simulink model "RobustAdaptive_Control"  (R2022b)
settings: Solver=VariableStepAuto  StartTime=0.0  StopTime=60  RelTol=1e-3
settings Model: Creator=JianFongLee  LastModifiedBy=allen
settings DebuggingCC: UnconnectedInputMsg=warning  UnconnectedOutputMsg=warning  UnconnectedLineMsg=warning
settings ModelReferenceCC: EnableRefExpFcnMdlSchedulingChecks=on
settings RTWCC: DLArmComputeVersion=19.05

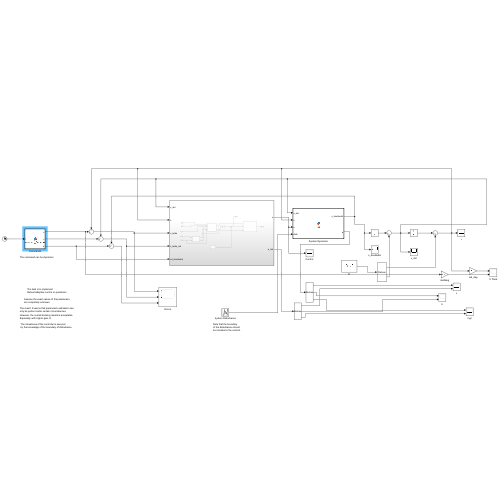
[thumbnail: Simulink's stored preview of the top-level diagram]
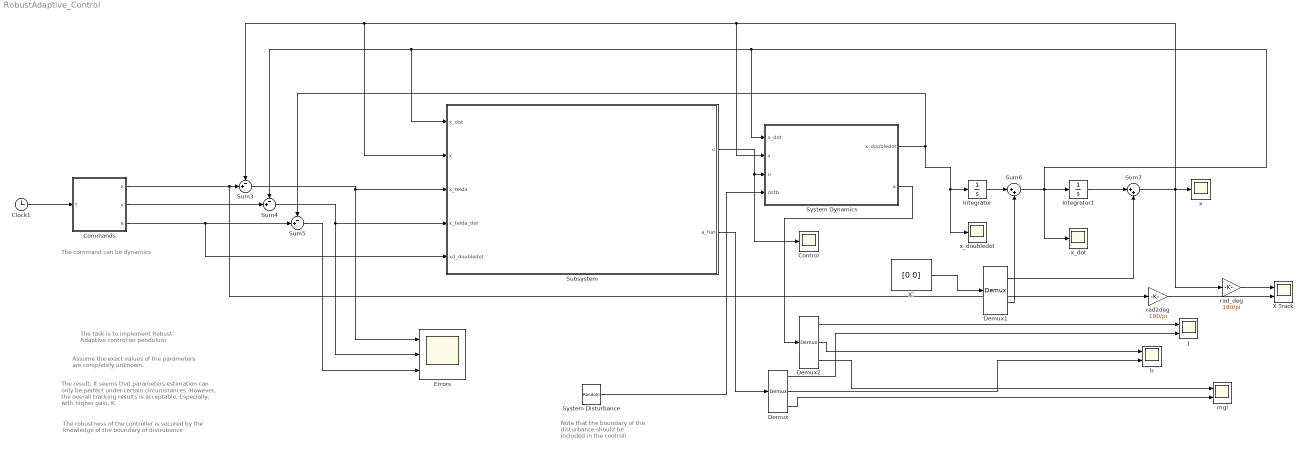
== system RobustAdaptive_Control ==
  note: The command can be dynamics
  note: The robustness of the controller is secured
      | by the knowledge of the boundary of distrubance
  note: Note that the boundary
      | of the disturbance should
      | be included in the controll.
  note: The result: It seems that parameters estimation can
      | only be perfect under certain circumstances.
      | However, the overall tracking results is acceptable.
      | Especially, with higher gain, K.
  note: Assume the exact values of the parameters
      | are completely unknown.
  note: The task is to implement
      | Robust Adaptive control on pendulum
  Clock1 : Clock
  Commands : MATLAB Function  TreatAsAtomicUnit=on
  Control : Scope
  Demux : Demux  Outputs=3
      settings: DisplayOption=none
  Demux1 : Demux  Outputs=2
      settings: DisplayOption=none
  Demux2 : Demux  Outputs=3
      settings: DisplayOption=none
  Errors : Scope  NumInputPorts=3
  IC : Constant  Value=[0 0]
  Integrator : Integrator
  Integrator1 : Integrator
  J : Scope  NumInputPorts=2
  Subsystem : Subsystem
  Sum3 : Sum  Inputs=-+|
  Sum4 : Sum  Inputs=-+|
  Sum5 : Sum  Inputs=-+|
  Sum6 : Sum  Inputs=|++
  Sum7 : Sum  Inputs=|++
  System Disturbance : UniformRandomNumber  Minimum=-2  Maximum=2  Seed=7
  System Dynamics : MATLAB Function  TreatAsAtomicUnit=on
  X Track : Scope  NumInputPorts=2
  b : Scope  NumInputPorts=2
  mgl : Scope  NumInputPorts=2
  rad2deg : Gain  Gain=180/pi
  rad_deg : Gain  Gain=180/pi
  x : Scope
  x_dot : Scope
  x_doubledot : Scope
  wires:
  Subsystem/1(u) -> Control/1, System Dynamics/3(u)
  IC/1 -> Demux1/1
  Integrator1/1 -> Sum7/1
  Integrator/1 -> Sum6/1
  Demux1/2 -> Sum6/2
  Sum6/1 -> x_dot/1, Subsystem/1(x_dot), Sum4/1, System Dynamics/1(x_dot), Integrator1/1
  Demux1/1 -> Sum7/2
  Sum7/1 -> rad_deg/1, Subsystem/2(x), Sum3/1, System Dynamics/2(x), x/1
  System Dynamics/1(x_doubledot) -> x_doubledot/1, Integrator/1, Sum5/1
  Sum3/1 -> Errors/1, Subsystem/3(x_telda)
  Sum4/1 -> Subsystem/4(x_telda_dot), Errors/2
  Clock1/1 -> Commands/1(t)
  Commands/1(x) -> rad2deg/1, Sum3/2
  Commands/2(v) -> Sum4/2
  Commands/3(a) -> Subsystem/5(xd_doubledot), Sum5/2
  Sum5/1 -> Errors/3
  Subsystem/2(a_hat) -> Demux/1
  System Dynamics/2(a) -> Demux2/1
  Demux2/1 -> J/1
  Demux/1 -> J/2
  Demux2/2 -> b/1
  Demux/2 -> b/2
  Demux2/3 -> mgl/1
  Demux/3 -> mgl/2
  rad_deg/1 -> X Track/1
  rad2deg/1 -> X Track/2
  System Disturbance/1 -> System Dynamics/4(dstb)

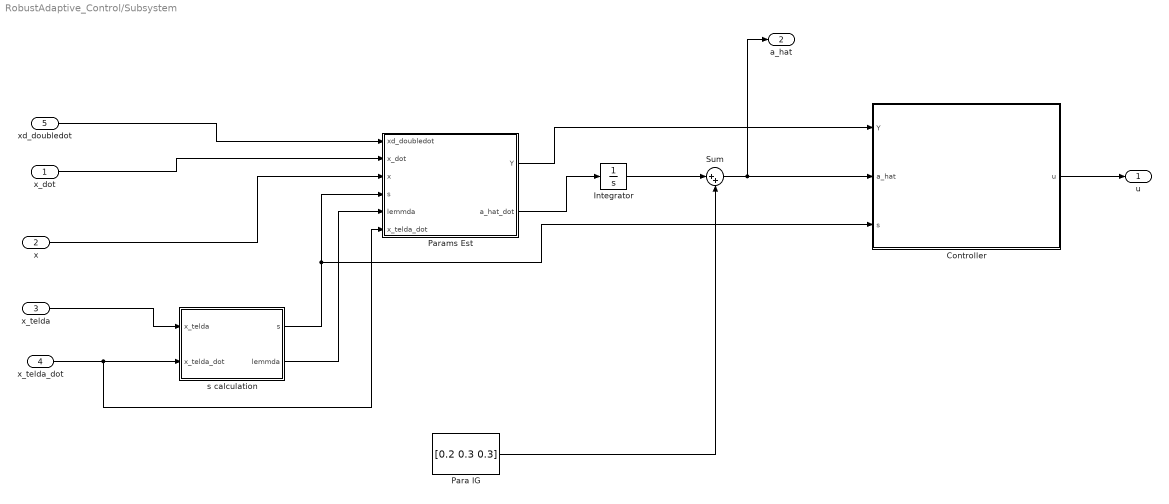
== system RobustAdaptive_Control/Subsystem ==
  x_dot : Inport
  x : Inport  Port=2
  x_telda : Inport  Port=3
  x_telda_dot : Inport  Port=4
  xd_doubledot : Inport  Port=5
  Controller : MATLAB Function  TreatAsAtomicUnit=on
  Integrator : Integrator
  Para IG : Constant  Value=[0.2 0.3 0.3]
  Params Est : MATLAB Function  TreatAsAtomicUnit=on
  Sum : Sum  Inputs=|++
  s calculation : MATLAB Function  TreatAsAtomicUnit=on
  u : Outport  OutDataTypeStr=double  PortDimensions=1
  a_hat : Outport  Port=2
  wires:
  x_telda/1 -> s calculation/1(x_telda)
  x_telda_dot/1 -> Params Est/6(x_telda_dot), s calculation/2(x_telda_dot)
  s calculation/1(s) -> Controller/3(s), Params Est/4(s)
  x/1 -> Params Est/3(x)
  x_dot/1 -> Params Est/2(x_dot)
  xd_doubledot/1 -> Params Est/1(xd_doubledot)
  Params Est/2(a_hat_dot) -> Integrator/1
  Params Est/1(Y) -> Controller/1(Y)
  s calculation/2(lemmda) -> Params Est/5(lemmda)
  Controller/1(u) -> u/1
  Integrator/1 -> Sum/1
  Para IG/1 -> Sum/2
  Sum/1 -> a_hat/1, Controller/2(a_hat)

== matlab function RobustAdaptive_Control/Subsystem/s calculation ==
  data: x_telda input; x_telda_dot input; s output; lemmda output
function [s,lemmda]= S(x_telda,x_telda_dot)
%%% Parameters Define
lemmda = 5.3;%%%should be greater than 0
s = x_telda_dot + lemmda*x_telda;
end

== matlab function RobustAdaptive_Control/Subsystem/Params Est ==
  data: Y output; xd_doubledot input; a_hat_dot output; x_dot input; x input; s input; lemmda input; x_telda_dot input
function [Y,a_hat_dot]= fcn(xd_doubledot,x_dot,x,s,lemmda,x_telda_dot)
%%% Parameters Defind
P = diag([2 2 0.3]);  %%% Postive Diagnoal
Uno = xd_doubledot + lemmda*x_telda_dot;
Dos = x_dot*abs(x_dot);
Tres = sin(x);

Y = [Uno Dos Tres];

a_hat_dot = s*Y*(P);

% a1_new = a_hat_dot(1);%%    J
% a2_new = a_hat_dot(2);%%    b
% a3_new = a_hat_dot(3);%%    mgl
end

== matlab function RobustAdaptive_Control/Subsystem/Controller ==
  data: Y input; a_hat input; u output; s input
function u = fcn(Y,a_hat,s)
%%% Parameters define
K = 5;    %%% K>0, 5 is the sweetspot,
          %%% and this value manefasts the importance of dstb supression
R = 50;     %%% Restriction
%%% K should be great enough for rapid tracking
c = 2;  %%% Should be consistent with sytem dynamics
if(s==0)    %%% Avoid singularity
    u = Y*a_hat;
else
     u = Y*a_hat + K*s + c*s/abs(s); 
     %u = Y*a_hat + K*s;
end

if(u>R)
    u = R;
elseif(u<-R)
    u = -R;
end

end

%%% Conclusion
%%% Line 11, with supression, the tracking converges faster

%%% Line 12, without supression, the tracking converges slower

== matlab function RobustAdaptive_Control/System Dynamics ==
  data: x_dot input; x input; u input; x_doubledot output; a output; dstb input
function [x_doubledot, a]= fcn(x_dot,x,u,dstb)
%%% System Parameters definition:
%%% J,b,mgl should be reasonable for a inverted pendulum
J = 5;
b = 2;
mgl = 7.5;
a = [J b mgl];  %%%output for visual comparision
%%% Dynamics Calculation
x_doubledot = (u - b*x_dot*abs(x_dot) - mgl*sin(x) - dstb)/J;
end

== matlab function RobustAdaptive_Control/Commands ==
  data: t input; x output; v output; a output
function [x,v,a]= Command_Generator(t)
%%% The function is to generate tracking commands for 
%%% the inverted pendulum problem

%%% Let the pendulum ocillates near upper eq point
%%% Parameters Define:
freq = 0.1;
omega = 2*pi*freq;
A = 0.1*pi;
%%% Command
%%% Sinusoidal Command
x = pi + A*sin(omega*t);
v = A*omega*cos(omega*t);
a = -A*(omega^2)*sin(omega*t);

%%% Step Command
% x = pi;
% v = 0;
% a = 0;
end
